simulink model "modelo_de_ejemplo"  (R2020b)
settings: Solver=VariableStepAuto  StartTime=0.0  StopTime=10.0  RelTol=1e-3
settings Model: Creator=Aitor  LastModifiedBy=Aitor

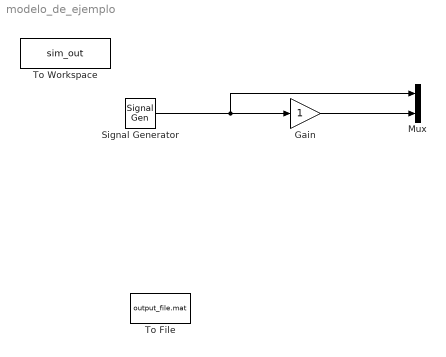
== system modelo_de_ejemplo ==
  Gain : Gain
  Mux : Mux  Inputs=2
  Signal Generator : SignalGenerator  Amplitude=2
  To File : ToFile  Filename=output_file.mat
  To Workspace : ToWorkspace  VariableName=sim_out  SaveFormat=Structure With Time  SampleTime=-1
  wires:
  Signal Generator/1 -> Mux/1, Gain/1
  Gain/1 -> Mux/2
